simulink model "PMSMModel"  (R2016a)
settings: Solver=ode4  StartTime=0.0  StopTime=2  FixedStep=1e-04  RelTol=1e-3
libraries: powerlib x6
settings Model: Creator=B210b  LastModifiedBy=B210b

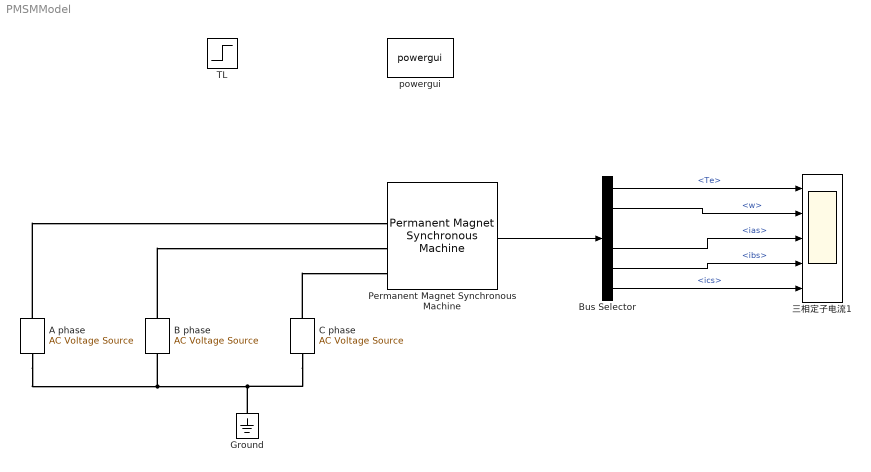
== system PMSMModel ==
  A phase : powerlib/Electrical Sources/AC Voltage Source  Amplitude=220*sqrt(2)  Phase=0  Frequency=50  SampleTime=0  Measurements=None  BusType=swing  Pref=10e3  Qref=0  Qmin=-inf  Qmax=+inf
  B phase : powerlib/Electrical Sources/AC Voltage Source  Amplitude=220*sqrt(2)  Phase=120  Frequency=50  SampleTime=0  Measurements=None  BusType=swing  Pref=10e3  Qref=0  Qmin=-inf  Qmax=+inf
  Bus Selector : BusSelector  OutputSignals=Te,w,theta,ias,ibs,ics
  C phase : powerlib/Electrical Sources/AC Voltage Source  Amplitude=220*sqrt(2)  Phase=-120  Frequency=50  SampleTime=0  Measurements=None  BusType=swing  Pref=10e3  Qref=0  Qmin=-inf  Qmax=+inf
  Ground : powerlib/Elements/Ground  LConnTagsString=a
  Permanent Magnet Synchronous Machine : powerlib/Machines/Permanent Magnet Synchronous Machine  NbPhases=3  FluxDistribution=Sinusoidal  RotorType=Round  MechanicalLoad=Torque Tm  PresetModel=No  ShowDetailedParameters=on  MeasurementBus=on  Resistance=0.22  Inductance=8.5e-3  dqInductances=[0.005 0.005]  La=0.005  MachineConstant=Flux linkage established by magnets (V.s)  Flux=0.117333  VoltageCst=106.4093  TorqueCst=0.88  Flat=120  Mechanical=[0.000624 0.000303448 5]  PolePairs=4  InitialConditions=[0,0, 0,0]  InitialConditions5ph=[0 0 0 0 0 0]  TsPowergui=0  TsBlock=-1  RefAngle=Aligned with phase A axis (original Park)
  TL : Step  Time=0.2  After=10  SampleTime=0
  powergui : powerlib/powergui  Priority=1  SimulationMode=Continuous  SolverType=Tustin/Backward Euler (TBE)  SampleTime=1e-4  frequency=60  SPID=off  DisableSnubberDevices=off  DisableRonSwitches=off  DisableVfSwitches=off  SwTol=0  DisplayEquations=off  Interpol=off  ExternalGateDelay=off  methode=off  Ts=10  FunctionMessages=off  echomessages=off  HookPort=off  EnableUseOfTLC=off  x0status=blocks  frequencyindice=0  Pbase=100e6  ErrMax=1e-4  Iterations=50  UnitsV=kV  UnitsW=MW  buscounter=0  RestoreLinks=warning  ResistiveCurrentMeasurement=off  Frange=[0:2:500]  Ylog=off  Xlog=on  ShowGrid=off  save=off  variable=ZData  structure=0  ZoomFFT=off  StartTime=0.0  cycles=1  DisplayStyle=1  fundamental=60  FreqAxis=off  MaxFrequency=1000  frequencyindicesteady=1  RmsSteady=1  display=off
  三相定子电流1 : Scope  NumInputPorts=5
  wires:
  Permanent Magnet Synchronous Machine/1 -> Bus Selector/1
  Bus Selector/1 -> 三相定子电流1/1  "<Te>"
  Bus Selector/2 -> 三相定子电流1/2  "<w>"
  Bus Selector/4 -> 三相定子电流1/3  "<ias>"
  Bus Selector/5 -> 三相定子电流1/4  "<ibs>"
  Bus Selector/6 -> 三相定子电流1/5  "<ics>"
  connections:
  A phase/RConn1 -- Permanent Magnet Synchronous Machine/LConn1
  B phase/RConn1 -- Permanent Magnet Synchronous Machine/LConn2
  A phase/LConn1 -- C phase/LConn1 -- Ground/LConn1 -- B phase/LConn1
  C phase/RConn1 -- Permanent Magnet Synchronous Machine/LConn3
